simulink model "SpeedModesControl_V2"  (R2022a)
settings: Solver=VariableStepAuto  StartTime=0.0  StopTime=10.0  RelTol=1e-3
libraries: simulink x6
settings Model: Creator=mluser  LastModifiedBy=mluser

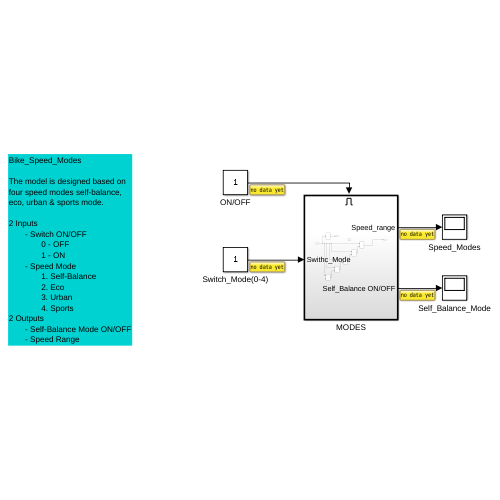
[thumbnail: Simulink's stored preview of the top-level diagram]
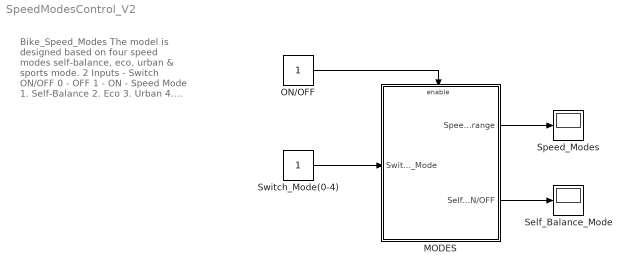
== system SpeedModesControl_V2 ==
  note: Bike_Speed_Modes
      |
      | The model is designed based on
      | four speed modes self-balance,
      | eco, urban & sports mode.
      |
      | 2 Inputs
      | 	- Switch ON/OFF
      | 		0 - OFF
      | 		1 - ON
      | 	- Speed Mode
      | 		1. Self-Balance
      | 		2. Eco
      | 		3. Urban
      | 		4. Sports
      | 2 Outputs
      | 	- Self-Balance Mode ON/OFF
      | 	- Speed Range
  MODES : Subsystem
  ON/OFF : Constant
  Self_Balance_Mode : Display
  Speed_Modes : Display
  Switch_Mode(0-4) : Constant
  wires:
  Switch_Mode(0-4)/1 -> MODES/1(Swithc_Mode)
  MODES/1(Speed_range) -> Speed_Modes/1
  MODES/2(Self_Balance ON/OFF) -> Self_Balance_Mode/1
  ON/OFF/1 -> MODES/Enable

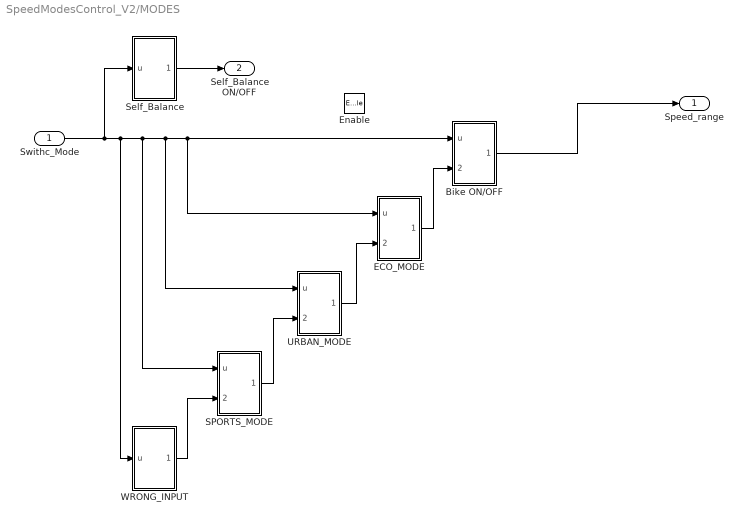
== system SpeedModesControl_V2/MODES ==
  Swithc_Mode : Inport
  Enable : EnablePort
  Bike ON/OFF : Subsystem
  ECO_MODE : Subsystem
  SPORTS_MODE : Subsystem
  Self_Balance : Subsystem
  URBAN_MODE : Subsystem
  WRONG_INPUT : Subsystem
  Speed_range : Outport
  Self_Balance ON/OFF : Outport  Port=2
  wires:
  Swithc_Mode/1 -> Bike ON/OFF/1(u), ECO_MODE/1(u), URBAN_MODE/1(u), SPORTS_MODE/1(u), WRONG_INPUT/1(u), Self_Balance/1(u)
  Self_Balance/1(Out1) -> Self_Balance ON/OFF/1
  Bike ON/OFF/1(Out1) -> Speed_range/1
  ECO_MODE/1(Out1) -> Bike ON/OFF/2(In2)
  URBAN_MODE/1(Out1) -> ECO_MODE/2(In2)
  SPORTS_MODE/1(Out1) -> URBAN_MODE/2(In2)
  WRONG_INPUT/1(Out1) -> SPORTS_MODE/2(In2)

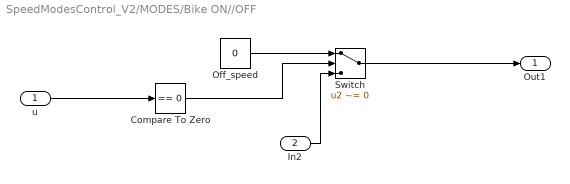
== system SpeedModesControl_V2/MODES/Bike ON//OFF ==
  u : Inport
  In2 : Inport  Port=2
  Compare To Zero : simulink/Logic and Bit Operations/Compare To Zero  relop===  OutDataTypeStr=boolean
  Off_speed : Constant  Value=0
  Switch : Switch  Criteria=u2 ~= 0  SaturateOnIntegerOverflow=off  InputSameDT=off
  Out1 : Outport
  wires:
  Compare To Zero/1 -> Switch/2
  Switch/1 -> Out1/1
  Off_speed/1 -> Switch/1
  In2/1 -> Switch/3
  u/1 -> Compare To Zero/1

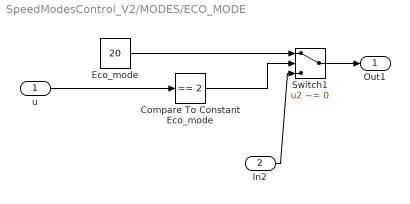
== system SpeedModesControl_V2/MODES/ECO_MODE ==
  u : Inport
  In2 : Inport  Port=2
  Compare To Constant Eco_mode : simulink/Logic and Bit Operations/Compare To Constant  relop===  const=2  OutDataTypeStr=boolean
  Eco_mode : Constant  Value=20
  Switch1 : Switch  Criteria=u2 ~= 0  SaturateOnIntegerOverflow=off  InputSameDT=off
  Out1 : Outport
  wires:
  Eco_mode/1 -> Switch1/1
  Compare To Constant Eco_mode/1 -> Switch1/2
  Switch1/1 -> Out1/1
  u/1 -> Compare To Constant Eco_mode/1
  In2/1 -> Switch1/3

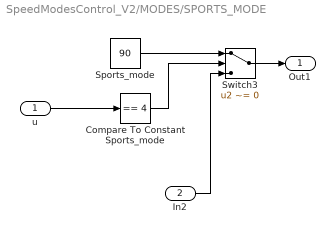
== system SpeedModesControl_V2/MODES/SPORTS_MODE ==
  u : Inport
  In2 : Inport  Port=2
  Compare To Constant Sports_mode : simulink/Logic and Bit Operations/Compare To Constant  relop===  const=4  OutDataTypeStr=boolean
  Sports_mode : Constant  Value=90
  Switch3 : Switch  Criteria=u2 ~= 0  SaturateOnIntegerOverflow=off  InputSameDT=off
  Out1 : Outport
  wires:
  Compare To Constant Sports_mode/1 -> Switch3/2
  Sports_mode/1 -> Switch3/1
  Switch3/1 -> Out1/1
  In2/1 -> Switch3/3
  u/1 -> Compare To Constant Sports_mode/1

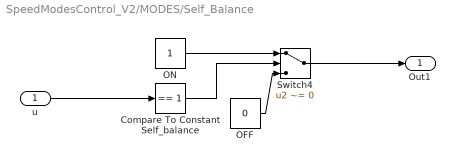
== system SpeedModesControl_V2/MODES/Self_Balance ==
  u : Inport
  Compare To Constant Self_balance : simulink/Logic and Bit Operations/Compare To Constant  relop===  const=1  OutDataTypeStr=boolean
  OFF : Constant  Value=0
  ON : Constant
  Switch4 : Switch  Criteria=u2 ~= 0  SaturateOnIntegerOverflow=off  InputSameDT=off
  Out1 : Outport
  wires:
  OFF/1 -> Switch4/3
  ON/1 -> Switch4/1
  Compare To Constant Self_balance/1 -> Switch4/2
  Switch4/1 -> Out1/1
  u/1 -> Compare To Constant Self_balance/1

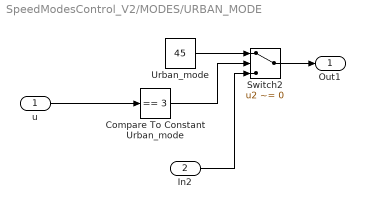
== system SpeedModesControl_V2/MODES/URBAN_MODE ==
  u : Inport
  In2 : Inport  Port=2
  Compare To Constant Urban_mode : simulink/Logic and Bit Operations/Compare To Constant  relop===  const=3  OutDataTypeStr=boolean
  Switch2 : Switch  Criteria=u2 ~= 0  SaturateOnIntegerOverflow=off  InputSameDT=off
  Urban_mode : Constant  Value=45
  Out1 : Outport
  wires:
  Switch2/1 -> Out1/1
  Compare To Constant Urban_mode/1 -> Switch2/2
  Urban_mode/1 -> Switch2/1
  u/1 -> Compare To Constant Urban_mode/1
  In2/1 -> Switch2/3

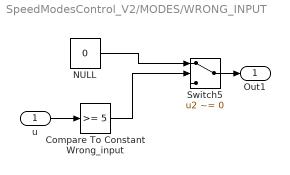
== system SpeedModesControl_V2/MODES/WRONG_INPUT ==
  u : Inport
  Compare To Constant Wrong_input : simulink/Logic and Bit Operations/Compare To Constant  relop=>=  const=5  OutDataTypeStr=boolean
  NULL : Constant  Value=0
  Switch5 : Switch  Criteria=u2 ~= 0  SaturateOnIntegerOverflow=off  InputSameDT=off
  Out1 : Outport
  wires:
  Compare To Constant Wrong_input/1 -> Switch5/2
  NULL/1 -> Switch5/1
  u/1 -> Compare To Constant Wrong_input/1
  Switch5/1 -> Out1/1
